simulink model "DM"  (R2023b)
settings: Solver=VariableStepAuto  StartTime=0.0  StopTime=10.0  RelTol=1e-3
libraries: dspquant2 x2, dspfdesign x1
settings Model: Creator=maruv  LastModifiedBy=maruv

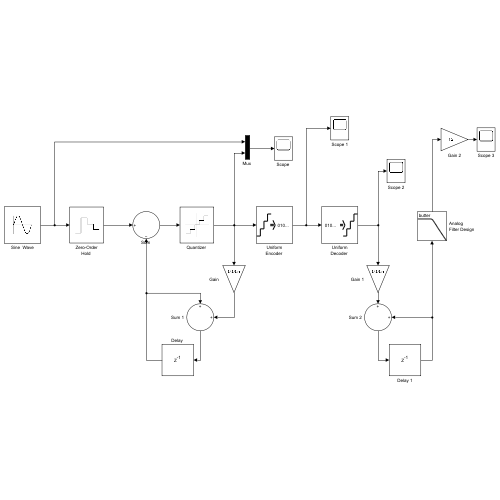
[thumbnail: Simulink's stored preview of the top-level diagram]
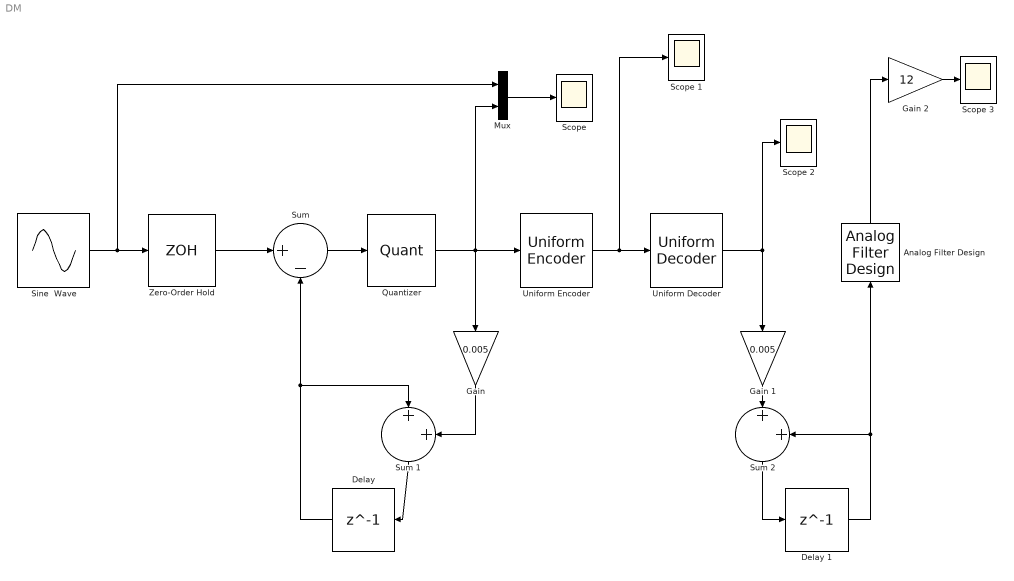
== system DM ==
  "Analog Filter Design " : dspfdesign/Analog Filter Design  method=Butterworth  filttype=Lowpass  N=8  Wlo=2*pi*100  Whi=80  Rp=2  Rs=40
  "Delay " : Delay  DelayLength=1  InitialCondition=0
  Delay 1 : Delay  DelayLength=1  InitialCondition=0
  "Gain " : Gain  Gain=0.005
  Gain 1 : Gain  Gain=0.005
  Gain 2 : Gain  Gain=12
  "Mux " : Mux  Inputs=2
  "Quantizer " : Quantizer
  Scope {,1..3} (4 alike) : Scope
  Sine  Wave : Sin  Amplitude=1.5  Frequency=2*pi*80  SampleTime=0
  "Sum " : Sum  Inputs=|+-
  Sum 1 : Sum  Inputs=|++
  Sum 2 : Sum  Inputs=|++
  "Uniform Decoder " : dspquant2/Uniform Decoder  peak=2  bits=8  overflowMode=Saturate  otype=Double
  "Uniform Encoder " : dspquant2/Uniform Encoder  peak=2  bits=8  otype=Unsigned integer
  "Zero-Order Hold " : ZeroOrderHold  SampleTime=1/8000
  wires:
  Sine  Wave/1 -> "Mux "/1, "Zero-Order Hold "/1
  "Zero-Order Hold "/1 -> "Sum "/1
  "Sum "/1 -> "Quantizer "/1
  "Quantizer "/1 -> "Uniform Encoder "/1, "Gain "/1, "Mux "/2
  Sum 1/1 -> "Delay "/1
  "Gain "/1 -> Sum 1/2
  "Delay "/1 -> Sum 1/1, "Sum "/2
  Gain 1/1 -> Sum 2/1
  "Uniform Encoder "/1 -> Scope 1/1, "Uniform Decoder "/1
  "Uniform Decoder "/1 -> Scope 2/1, Gain 1/1
  Sum 2/1 -> Delay 1/1
  Delay 1/1 -> Sum 2/2, "Analog Filter Design "/1
  "Analog Filter Design "/1 -> Gain 2/1
  "Mux "/1 -> "Scope "/1
  Gain 2/1 -> Scope 3/1
